simulink model "Mapped_SIengine"  (R2020a)
settings: Solver=ode45  StartTime=0.0  StopTime=inf  RelTol=1e-3
model workspace (MAT data in the model file):
  f_air = [0 0 0 0 0 0 0 0 0 0 0 0 ... (1600 elements, 40x40)]
  f_air_2 = [0 0 0 0 0 0 0 0 0 0 0 0 ... (1600 elements, 40x40)]
  f_air_3 = [0 0 0 0 0 0 0 0 0 0 0 0 ... (1600 elements, 40x40)]
  f_co = [0 0 0 0 0 0 0 0 0 0 0 0 ... (1600 elements, 40x40)]
  f_co2 = [0 0 0 0 0 0 0 0 0 0 0 0 ... (1600 elements, 40x40)]
  f_co2_2 = [0 0 0 0 0 0 0 0 0 0 0 0 ... (1600 elements, 40x40)]
  f_co2_3 = [0 0 0 0 0 0 0 0 0 0 0 0 ... (1600 elements, 40x40)]
  f_co_2 = [0 0 0 0 0 0 0 0 0 0 0 0 ... (1600 elements, 40x40)]
  f_co_3 = [0 0 0 0 0 0 0 0 0 0 0 0 ... (1600 elements, 40x40)]
  f_eff = [670.316996187 720.308767781 792.957689567 866.984724439 936.107262509 993.6074505 1032.32016026 1045.96464526 1030.49338049 985.210416561 913.453890857 822.583118779 ... (1600 elements, 40x40)]
  f_eff_2 = [684.642644828 714.282646475 766.065877319 834.489440327 904.708162294 965.410962814 1008.68315654 1027.52605684 1017.26674508 976.676361151 908.692031431 820.456453525 ... (1600 elements, 40x40)]
  f_eff_3 = [1006.399029 988.985858566 966.191164384 942.942726285 919.13814889 894.633744735 869.224086827 842.609277842 814.34087126 783.729495015 749.683700315 710.445098186 ... (1600 elements, 40x40)]
  f_fuel = [0 0 0 0 0 0 0 0 0 0 0 0 ... (1600 elements, 40x40)]
  f_fuel_2 = [0 0 0 0 0 0 0 0 0 0 0 0 ... (1600 elements, 40x40)]
  f_fuel_3 = [0 0 0 0 0 0 0 0 0 0 0 0 ... (1600 elements, 40x40)]
  f_hc = [0 0 0 0 0 0 0 0 0 0 0 0 ... (1600 elements, 40x40)]
  f_hc_2 = [0 0 0 0 0 0 0 0 0 0 0 0 ... (1600 elements, 40x40)]
  f_hc_3 = [0 0 0 0 0 0 0 0 0 0 0 0 ... (1600 elements, 40x40)]
  f_nox = [0 0 0 0 0 0 0 0 0 0 0 0 ... (1600 elements, 40x40)]
  f_nox_2 = [0 0 0 0 0 0 0 0 0 0 0 0 ... (1600 elements, 40x40)]
  f_nox_3 = [0 0 0 0 0 0 0 0 0 0 0 0 ... (1600 elements, 40x40)]
  f_pm = [0 0 0 0 0 0 0 0 0 0 0 0 ... (1600 elements, 40x40)]
  f_pm_2 = [0 0 0 0 0 0 0 0 0 0 0 0 ... (1600 elements, 40x40)]
  f_pm_3 = [0 0 0 0 0 0 0 0 0 0 0 0 ... (1600 elements, 40x40)]
  f_tbrake = [0 1.249866 2.86153531579 4.47320463158 5 5 5 5 5 5 5 5 ... (1600 elements, 40x40)]
  f_tbrake_2 = [0 1.249866 2.86153531579 4.47320463158 5 5 5 5 5 5 5 5 ... (1600 elements, 40x40)]
  f_tbrake_3 = [0 1.249866 2.86153531579 4.47320463158 6.08487394737 7.69654326316 9.30821257895 10.9198818947 11.1629500974 11.1629500974 11.1629500974 11.1629500974 ... (1600 elements, 40x40)]
  f_tbrake_n_bpt = [0 0 263.157894737 526.315789474 789.473684211 1052.63157895 1315.78947368 1578.94736842 1842.10526316 2105.26315789 2368.42105263 2631.57894737 ... (40 elements, 40x1)]
  f_tbrake_n_bpt_2 = [0 0 263.157894737 526.315789474 789.473684211 1052.63157895 1315.78947368 1578.94736842 1842.10526316 2105.26315789 2368.42105263 2631.57894737 ... (40 elements, 40x1)]
  f_tbrake_n_bpt_3 = [0 250 506.578947368 763.157894737 1019.73684211 1276.31578947 1532.89473684 1789.47368421 2046.05263158 2302.63157895 2559.21052632 2815.78947368 ... (40 elements, 40x1)]
  f_tbrake_t_bpt = [0 1.249866 2.86153531579 4.47320463158 6.08487394737 7.69654326316 9.30821257895 10.9198818947 12.5315512105 14.1432205263 15.7548898421 17.3665591579 ... (40 elements, 40x1)]
  f_tbrake_t_bpt_2 = [0 1.249866 2.86153531579 4.47320463158 6.08487394737 7.69654326316 9.30821257895 10.9198818947 12.5315512105 14.1432205263 15.7548898421 17.3665591579 ... (40 elements, 40x1)]
  f_tbrake_t_bpt_3 = [0 1.249866 2.86153531579 4.47320463158 6.08487394737 7.69654326316 9.30821257895 10.9198818947 12.5315512105 14.1432205263 15.7548898421 17.3665591579 ... (40 elements, 40x1)]
  f_texh = [293.009633718 294.857313146 297.052397084 299.699051886 302.858034892 306.451912682 310.462681698 314.882875816 319.709442503 324.946127175 330.611464251 336.7535529 ... (1600 elements, 40x40)]
  f_texh_2 = [289.156357026 292.232481099 295.694373493 298.759895612 302.078903236 305.825167361 309.967750743 314.502661641 319.430702614 324.756555872 330.499613015 336.708696186 ... (1600 elements, 40x40)]
  f_texh_3 = [268.493646048 274.583667898 282.390577341 290.134630796 297.801509677 305.3737657 312.830149781 320.145043025 327.288485306 334.228167231 340.936997934 347.415144896 ... (1600 elements, 40x40)]
undefined symbols (not defined in the file): maxtrq
libraries: autolibsharedmappedengines x1
(part 4 of 4)

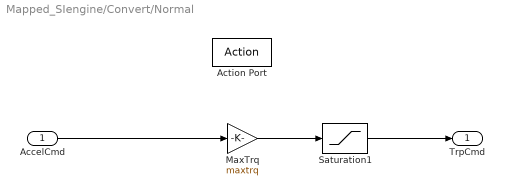
== system Mapped_SIengine/Convert/Normal ==
  AccelCmd : Inport
  Action Port : ActionPort
  MaxTrq : Gain  Gain=maxtrq
  Saturation1 : Saturate  UpperLimit=1  LowerLimit=0
  TrpCmd : Outport
  wires:
  Saturation1/1 -> TrpCmd/1
  AccelCmd/1 -> MaxTrq/1
  MaxTrq/1 -> Saturation1/1

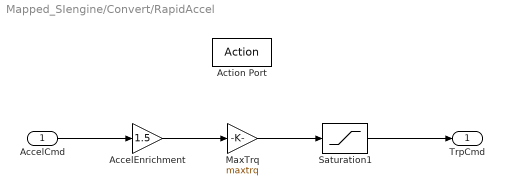
== system Mapped_SIengine/Convert/RapidAccel ==
  AccelCmd : Inport
  Action Port : ActionPort
  "AccelEnrichment " : Gain  Gain=1.5
  MaxTrq : Gain  Gain=maxtrq
  Saturation1 : Saturate  UpperLimit=1  LowerLimit=0
  TrpCmd : Outport
  wires:
  MaxTrq/1 -> Saturation1/1
  "AccelEnrichment "/1 -> MaxTrq/1
  AccelCmd/1 -> "AccelEnrichment "/1
  Saturation1/1 -> TrpCmd/1

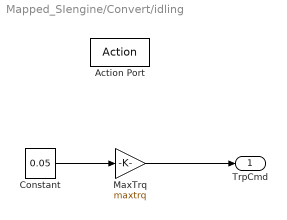
== system Mapped_SIengine/Convert/idling ==
  Action Port : ActionPort
  Constant : Constant  Value=0.05
  MaxTrq : Gain  Gain=maxtrq
  TrpCmd : Outport
  wires:
  Constant/1 -> MaxTrq/1
  MaxTrq/1 -> TrpCmd/1
